simulink model "Elicottero_fuori"  (R2026a)
settings: Solver=VariableStepAuto
values from neighbouring files (symbols this model uses):
  c_alpha = 0.01    [Params_Progetto.m]    (also in Params_Progetto_master.m; parameters.m; parameters_parametrico.m)
  c_beta = 0.01    [Params_Progetto.m]    (also in Params_Progetto_master.m; parameters.m; parameters_parametrico.m)
  eps_p = 0.1    [Params_Progetto.m]    (also in Params_Progetto_master.m; parameters.m; parameters_parametrico.m)
  eps_y = 0.1    [Params_Progetto.m]    (also in Params_Progetto_master.m; parameters.m; parameters_parametrico.m)
  g = 9.81    [Params_Progetto.m]    (also in Params_Progetto_master.m; parameters.m; parameters_parametrico.m)
  h0 = 0.30    (= 0.3)    [Params_Progetto.m]    (also in Params_Progetto_master.m)
  I_b = 0.00023    [Params_Progetto.m]    (also in Params_Progetto_master.m; parameters.m; parameters_parametrico.m)
  J_alpha = 0.012    [Params_Progetto.m]    (also in Params_Progetto_master.m; parameters.m; parameters_parametrico.m)
  J_y = 0.00023    [Params_Progetto.m]    (also in Params_Progetto_master.m; parameters.m; parameters_parametrico.m)
  J_z = 0.00364    [Params_Progetto.m]    (also in Params_Progetto_master.m; parameters.m; parameters_parametrico.m)
  l = 0.2    [Params_Progetto.m]    (also in Params_Progetto_master.m; parameters.m; parameters_parametrico.m)
  m = 0.2    [Params_Progetto.m]    (also in Params_Progetto_master.m; parameters.m; parameters_parametrico.m)
  P0_EKF = diag([ ... (first row only)    [Params_Progetto.m]    (also in Params_Progetto_master.m; parameters.m = diag([1, 1, 1, 1]); parameters_parametrico.m = diag([10, 10, 10, 10]))
  Q_EKF = diag([ ... (first row only)    [Params_Progetto.m]    (also in Params_Progetto_master.m; parameters.m = diag([1e-6, 1e-4, 1e-6, 1e-4]); parameters_parametrico.m = diag([1e-5, 1e-3, 1e-5, 1e-3]))
  R_EKF = diag([ ... (first row only)    [Params_Progetto.m]    (also in Params_Progetto_master.m; parameters.m = diag([std_dev_cam^2, std_dev_cam^2, std_dev_acc^2]); parameters_parametrico.m)
  sigma_acc_sensor = 0.05    [Params_Progetto.m]    (also in Params_Progetto_master.m)
  sigma_alpha_sensor = 0.01    [Params_Progetto.m]    (also in Params_Progetto_master.m)
  sigma_cam_sensor = 0.002    [Params_Progetto.m]    (also in Params_Progetto_master.m = 0.005)
  Ts_Acceler = 1 / 80    (= 0.0125)    [Params_Progetto.m]    (also in Params_Progetto_master.m)
  Ts_EKF = 1/104    (= 0.00961538461538)    [Params_Progetto.m]    (also in Params_Progetto_master.m)
  Ts_ToF_alpha = 1 / 30    (= 0.0333333333333)    [Params_Progetto.m]    (also in Params_Progetto_master.m)
  Ts_Tof_cam = 1/45    (= 0.0222222222222)    [Params_Progetto.m]    (also in Params_Progetto_master.m)
  x0_EKF = [0; 0; 0; 0]    [Params_Progetto.m]    (also in Params_Progetto_master.m; parameters.m; parameters_parametrico.m = [pi/2; 0.2; pi/4; -0.15])
libraries: simulink x2
settings Model: Creator=filin  LastModifiedBy=tomma

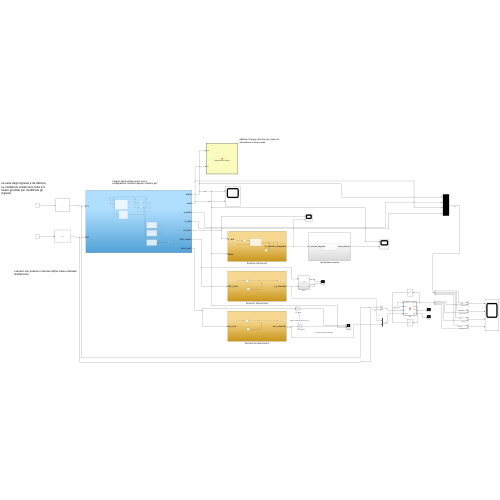
[thumbnail: Simulink's stored preview of the top-level diagram]
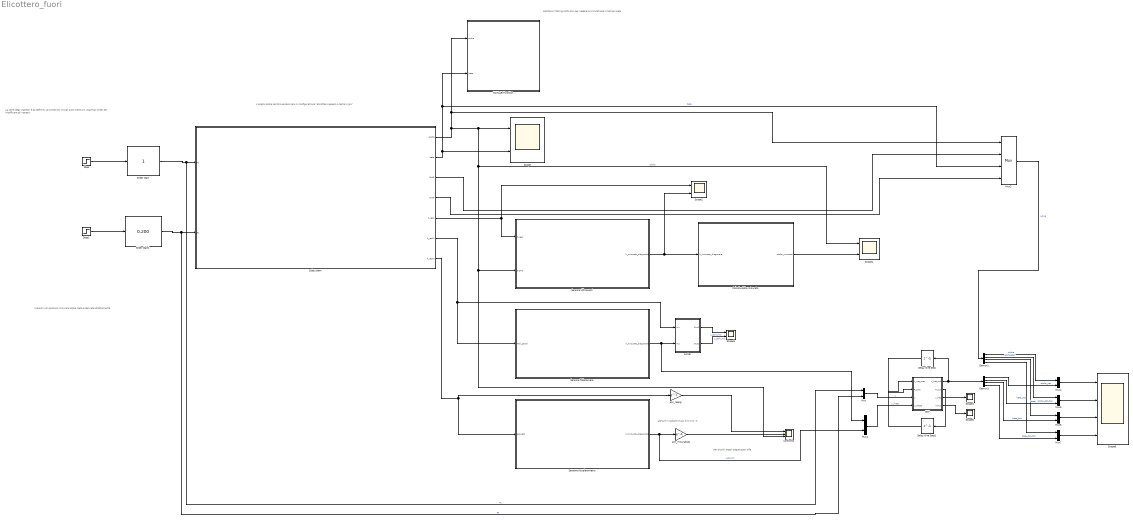
== system Elicottero_fuori ==
  note: alpha è in radianti e acc è in m/s^2
  note: per piccoli angoli segue quasi alfa
  note: L'angolo alpha sembra essere zero in configurazione "elicottero appeso a testa in giù"
  note: Abilitare il Pacing sotto Run per vedere la simulazione in tempo reale
  note: I sensori non possono misurare alpha, beta e derivate direttamente
  note: La serie degli ingressi è da definire,
      | Le condizioni iniziali sono tutte a 0. Usare gli slider per modificare gli ingressi
  Calcola alpha misurato : Subsystem
  Delay One Step : Delay  DelayLength=1  InitialCondition=x0_EKF  SampleTime=Ts_EKF
  Delay One Step1 : Delay  DelayLength=1  InitialCondition=P0_EKF  SampleTime=Ts_EKF
  Demux2 : Demux
  Demux3 : Demux
  EKF : MATLAB Function  TreatAsAtomicUnit=on
  MATLAB Function : MATLAB Function  TreatAsAtomicUnit=on
  Mux{,1,4..7} (6 alike) : Mux  Inputs=2
  Mux2 : Mux
  Scope{,1..3} (4 alike) : Scope  NumInputPorts=2
      Scope settings: ActiveDisplayYMinimum=-0.63060301461050317  ActiveDisplayYMaximum=0.90405934016402656
      Scope1 settings: ActiveDisplayYMinimum=0.070707009259759535  ActiveDisplayYMaximum=0.469619980054257
      Scope2 settings: ActiveDisplayYMinimum=0.074242701385080767  ActiveDisplayYMaximum=0.48624550790168564  DataLoggingVariableName=ScopeData2
      Scope3 settings: ActiveDisplayYMinimum=0.097019421313557869  ActiveDisplayYMaximum=0.17329990637736653  DataLoggingVariableName=ScopeData3
  Scope4 : Scope
      settings: ActiveDisplayYMinimum=-0.80524166083087523  ActiveDisplayYMaximum=1.1715327148927259  DataLoggingVariableName=ScopeData5
  Scope5 : Scope
      settings: ActiveDisplayYMinimum=-0.57698730443451041  ActiveDisplayYMaximum=0.48376451557036515  DataLoggingVariableName=ScopeData6
  Scope6 : Scope  NumInputPorts=4
      settings: ActiveDisplayYMinimum=-0.81874656324729156  ActiveDisplayYMaximum=1.168245552270631  DataLoggingVariableName=ScopeData8
  Sensore Accelerometro : Subsystem
  Sensore Telecamera : Subsystem
  Sensore Ultrasuoni : Subsystem
  Slider Gain : simulink/Math Operations/Slider Gain  gain=1  low=0  high=4
  Slider Gain1 : simulink/Math Operations/Slider Gain  gain=0.200  low=-1  high=1
  Step : Step  InitialValue=1  FinalValue=0  SampleTime=0
  Step1 : Step  InitialValue=1  FinalValue=0  SampleTime=0
  Subsystem : Subsystem
  acc_misurato/g : Gain  Gain=g^-1
  acc_real/g : Gain  Gain=g^-1
  confronto : Scope  NumInputPorts=3
      settings: ActiveDisplayYMinimum=-1.8843706187467704  ActiveDisplayYMaximum=3.0235830228592131  DataLoggingVariableName=ScopeData4
  sorter : Subsystem
  wires:
  Step1/1 -> Slider Gain1/1
  Slider Gain1/1 -> Mux/2, Subsystem/2(F2)  "F2"
  Step/1 -> Slider Gain/1
  Slider Gain/1 -> Mux/1, Subsystem/1(F1)  "F1"
  Subsystem/1(alpha) -> MATLAB Function/1(alpha), Mux2/1, Scope1/1, confronto/3, Sensore Ultrasuoni/2(alpha), Scope/1  "alpha"
  Subsystem/2(beta) -> MATLAB Function/2(beta), Mux2/3, Scope/2  "beta"
  Subsystem/5(h_real) -> Sensore Ultrasuoni/1(h_real), Scope2/1
  Sensore Ultrasuoni/1(h_misurato_diagonale) -> Scope2/2, Calcola alpha misurato/1(h_misurato_diagonale)
  Calcola alpha misurato/1(alpha_misurato) -> Scope1/2
  Subsystem/6(h_real1) -> Sensore Telecamera/1(Tail_coord), sorter/1(In1)
  Sensore Telecamera/1(h_misurato_diagonale) -> Mux1/1, sorter/2(In2)
  sorter/1(Out1) -> Scope3/1  "x_cam_mis"
  sorter/2(Out2) -> Scope3/2  "y_cam_mis"
  Sensore Accelerometro/1(h_misurato_diagonale) -> Mux1/2, acc_misurato/g/1  "acc_mis"
  Subsystem/7(h_real2) -> Sensore Accelerometro/1(acc_real), acc_real/g/1
  acc_real/g/1 -> confronto/1
  acc_misurato/g/1 -> confronto/2
  Delay One Step/1 -> EKF/1(x_hat_prev)
  EKF/2(P_out) -> Delay One Step1/1
  Delay One Step1/1 -> EKF/2(P_prev)
  Mux/1 -> EKF/3(u)  "u"
  Mux1/1 -> EKF/4(y_meas)  "y_meas"
  Subsystem/3(Out3) -> Mux2/2
  Subsystem/4(Out4) -> Mux2/4
  Mux2/1 -> Demux2/1  "x_true"
  EKF/4(innov) -> Scope5/1
  Mux5/1 -> Scope6/2
  Demux3/2 -> Mux5/2  "alpha_dot_hat"
  Demux3/4 -> Mux7/2  "beta_dot_hat"
  Demux2/4 -> Mux7/1  "beta_dot"
  Demux2/3 -> Mux6/1  "beta"
  EKF/1(x_hat_out) -> Demux3/1, Delay One Step/1
  Demux3/3 -> Mux6/2  "beta_hat"
  Demux2/1 -> Mux4/1  "alpha"
  Demux3/1 -> Mux4/2  "alpha_hat"
  Demux2/2 -> Mux5/1  "alpha_dot"
  Mux7/1 -> Scope6/4
  Mux6/1 -> Scope6/3
  Mux4/1 -> Scope6/1
  EKF/3(y_hat) -> Scope4/1

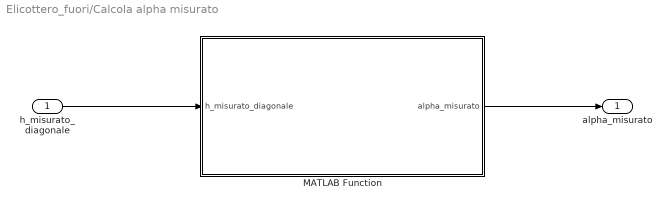
== system Elicottero_fuori/Calcola alpha misurato ==
  h_misurato_diagonale : Inport
  MATLAB Function : MATLAB Function  TreatAsAtomicUnit=on
  alpha_misurato : Outport
  wires:
  h_misurato_diagonale/1 -> MATLAB Function/1(h_misurato_diagonale)
  MATLAB Function/1(alpha_misurato) -> alpha_misurato/1

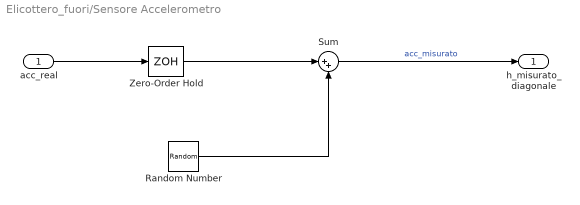
== system Elicottero_fuori/Sensore Accelerometro ==
  acc_real : Inport
  Random Number : RandomNumber  Variance=sigma_acc_sensor^2  Seed=1357  SampleTime=Ts_Acceler
  Sum : Sum  Inputs=|++
  Zero-Order Hold : ZeroOrderHold  SampleTime=Ts_Acceler
  h_misurato_diagonale : Outport
  wires:
  acc_real/1 -> Zero-Order Hold/1
  Zero-Order Hold/1 -> Sum/1
  Random Number/1 -> Sum/2
  Sum/1 -> h_misurato_diagonale/1  "acc_misurato"

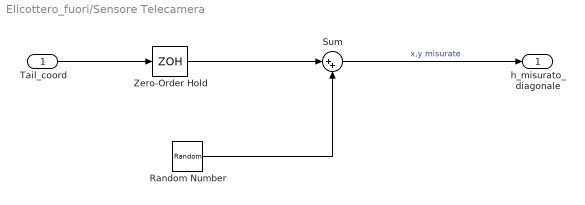
== system Elicottero_fuori/Sensore Telecamera ==
  Tail_coord : Inport
  Random Number : RandomNumber  Variance=sigma_cam_sensor^2  Seed=1357  SampleTime=Ts_Tof_cam
  Sum : Sum  Inputs=|++
  Zero-Order Hold : ZeroOrderHold  SampleTime=Ts_Tof_cam
  h_misurato_diagonale : Outport
  wires:
  Tail_coord/1 -> Zero-Order Hold/1
  Zero-Order Hold/1 -> Sum/1
  Random Number/1 -> Sum/2
  Sum/1 -> h_misurato_diagonale/1  "x,y misurate"

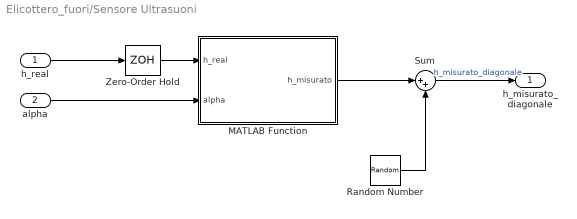
== system Elicottero_fuori/Sensore Ultrasuoni ==
  h_real : Inport
  alpha : Inport  Port=2
  MATLAB Function : MATLAB Function  TreatAsAtomicUnit=on
  Random Number : RandomNumber  Variance=sigma_alpha_sensor^2  Seed=1357  SampleTime=Ts_ToF_alpha
  Sum : Sum  Inputs=|++
  Zero-Order Hold : ZeroOrderHold  SampleTime=Ts_ToF_alpha
  h_misurato_diagonale : Outport
  wires:
  h_real/1 -> Zero-Order Hold/1
  Random Number/1 -> Sum/2
  Sum/1 -> h_misurato_diagonale/1  "h_misurato_diagonale"
  Zero-Order Hold/1 -> MATLAB Function/1(h_real)
  MATLAB Function/1(h_misurato) -> Sum/1
  alpha/1 -> MATLAB Function/2(alpha)

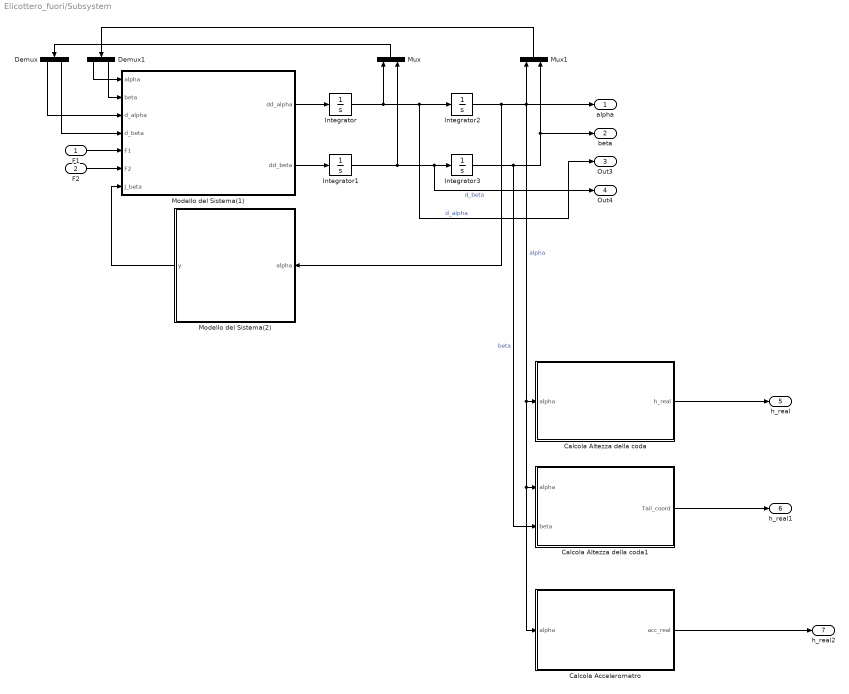
== system Elicottero_fuori/Subsystem ==
  F1 : Inport
  F2 : Inport  Port=2
  Calcola Accelerometro : MATLAB Function  TreatAsAtomicUnit=on
  Calcola Altezza della coda : MATLAB Function  TreatAsAtomicUnit=on
  Calcola Altezza della coda1 : MATLAB Function  TreatAsAtomicUnit=on
  Demux : Demux  Outputs=2
  Demux1 : Demux  Outputs=2
  Integrator : Integrator
  Integrator1 : Integrator
  Integrator2 : Integrator  WrapState=on
  Integrator3 : Integrator  WrapState=on
  Modello del Sistema(1) : MATLAB Function  TreatAsAtomicUnit=on
  Modello del Sistema(2) : MATLAB Function  TreatAsAtomicUnit=on
  Mux : Mux  Inputs=2
  Mux1 : Mux  Inputs=2
  alpha : Outport
  beta : Outport  Port=2
  Out3 : Outport  Port=3
  Out4 : Outport  Port=4
  h_real : Outport  Port=5
  h_real1 : Outport  Port=6
  h_real2 : Outport  Port=7
  wires:
  Demux1/2 -> Modello del Sistema(1)/2(beta)
  Integrator2/1 -> Modello del Sistema(2)/1(alpha), Calcola Accelerometro/1(alpha), Calcola Altezza della coda1/1(alpha), Calcola Altezza della coda/1(alpha), alpha/1, Mux1/1  "alpha"
  Integrator1/1 -> Mux/2, Out4/1, Integrator3/1  "d_beta"
  Mux/1 -> Demux/1
  Demux/2 -> Modello del Sistema(1)/4(d_beta)
  Modello del Sistema(2)/1(y) -> Modello del Sistema(1)/7(J_beta)
  Demux/1 -> Modello del Sistema(1)/3(d_alpha)
  Integrator3/1 -> beta/1, Mux1/2, Calcola Altezza della coda1/2(beta)  "beta"
  Modello del Sistema(1)/1(dd_alpha) -> Integrator/1
  Modello del Sistema(1)/2(dd_beta) -> Integrator1/1
  Demux1/1 -> Modello del Sistema(1)/1(alpha)
  Integrator/1 -> Mux/1, Out3/1, Integrator2/1  "d_alpha"
  Mux1/1 -> Demux1/1
  F2/1 -> Modello del Sistema(1)/6(F2)
  F1/1 -> Modello del Sistema(1)/5(F1)
  Calcola Altezza della coda/1(h_real) -> h_real/1
  Calcola Altezza della coda1/1(Tail_coord) -> h_real1/1
  Calcola Accelerometro/1(acc_real) -> h_real2/1

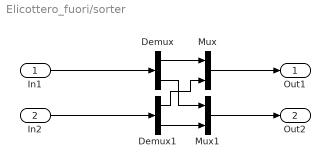
== system Elicottero_fuori/sorter ==
  In1 : Inport
  In2 : Inport  Port=2
  Demux : Demux  Outputs=2
  Demux1 : Demux  Outputs=2
  Mux : Mux  Inputs=2
  Mux1 : Mux  Inputs=2
  Out1 : Outport
  Out2 : Outport  Port=2
  wires:
  Demux/2 -> Mux1/1
  Demux/1 -> Mux/1
  Demux1/1 -> Mux/2
  In1/1 -> Demux/1
  Mux1/1 -> Out2/1
  In2/1 -> Demux1/1
  Demux1/2 -> Mux1/2
  Mux/1 -> Out1/1

== matlab function Elicottero_fuori/Subsystem/Calcola Accelerometro ==
  data: alpha input; acc_real output; g parameter
function acc_real = Compute_Accelerometer(alpha, g)

%%Si assume un accelerometro monoassiale solidale al corpo,
% orientato in modo da misurare la componente della gravità dovuta al pitch.

acc_real = g * sin(alpha);

%acc_real = -g * sin(alpha); quale usiamo?
end

== matlab function Elicottero_fuori/EKF ==
  data: x_hat_prev input; P_prev input; u input; x_hat_out output; y_meas input; P_out output; Ts_EKF parameter; Q_EKF parameter; R_EKF parameter; J_alpha parameter; J_y parameter; J_z parameter; I_b parameter; m parameter; l parameter; g parameter; c_alpha parameter; c_beta parameter; eps_p parameter; eps_y parameter; y_hat output; innov output
function [x_hat_out, P_out, y_hat, innov] = EKF(x_hat_prev, P_prev, u, y_meas, Ts_EKF, Q_EKF, R_EKF, J_alpha, J_y, J_z, I_b, m, l, g, c_alpha, c_beta, eps_p, eps_y)
% EKF
%
% Ingressi:
%   x_hat_prev = [alpha_hat; d_alpha_hat; beta_hat; d_beta_hat]
%   P_prev     = matrice 4x4 della covarianza precedente
%   u          = [F1; F2]
%   y_meas     = [x_cam_mis; y_cam_mis; acc_mis]
%
% Uscite:
%   x_hat_out  = stato corretto al passo corrente
%   P_out      = covarianza corretta al passo corrente

% ============================================================
% 1. Estrazione ingressi
% ============================================================

F1 = u(1);
F2 = u(2);

alpha   = x_hat_prev(1);
d_alpha = x_hat_prev(2);
beta    = x_hat_prev(3);
d_beta  = x_hat_prev(4);

% ============================================================
% 2. Modello dinamico continuo dell'elicottero
%    x_dot = f(x,u)
% ============================================================

J_beta = J_y*sin(alpha)^2 + (J_z + m*l^2)*cos(alpha)^2 + I_b;

dd_alpha = ( ...
    - c_alpha*d_alpha ...
    - m*g*l*sin(alpha) ...
    + l*F1*cos(beta) ...
    + eps_p*l*F2*sin(beta) ...
            ) / J_alpha;

dd_beta = ( ...
    - c_beta*d_beta ...
    + l*F2*cos(alpha) ...
    + eps_y*l*F1*sin(alpha) ...
          ) / J_beta;

f = [
    d_alpha;
    dd_alpha;
    d_beta;
    dd_beta
];

% ============================================================
% 3. Predizione discreta tramite Eulero
%    x(k|k-1) = x(k-1|k-1) + Ts*f(x,u)
% ============================================================

x_pred = x_hat_prev + Ts_EKF*f;

% ============================================================
% 4. Jacobiana continua A_c = df/dx
% ============================================================

Kgeom = J_z + m*l^2;

dJbeta_dalpha = 2*sin(alpha)*cos(alpha)*(J_y - Kgeom);

% Derivate di dd_alpha
d_ddalpha_d_alpha = -m*g*l*cos(alpha) / J_alpha;

d_ddalpha_d_dalpha = -c_alpha / J_alpha;

d_ddalpha_d_beta = ( ...
    -l*F1*sin(beta) ...
    + eps_p*l*F2*cos(beta) ...
    ) / J_alpha;

d_ddalpha_d_dbeta = 0;

% Derivate di dd_beta
N_beta = ...
    - c_beta*d_beta ...
    + l*F2*cos(alpha) ...
    + eps_y*l*F1*sin(alpha);

dNbeta_dalpha = ...
    - l*F2*sin(alpha) ...
    + eps_y*l*F1*cos(alpha);

d_ddbeta_d_alpha = ...
    (dNbeta_dalpha*J_beta - N_beta*dJbeta_dalpha) / (J_beta^2);

d_ddbeta_d_dalpha = 0;

d_ddbeta_d_beta = 0;

d_ddbeta_d_dbeta = -c_beta / J_beta;

A_c = [
    0,                 1,                  0,                0;
    d_ddalpha_d_alpha, d_ddalpha_d_dalpha, d_ddalpha_d_beta, d_ddalpha_d_dbeta;
    0,                 0,                  0,                1;
    d_ddbeta_d_alpha,  d_ddbeta_d_dalpha,  d_ddbeta_d_beta,  d_ddbeta_d_dbeta
];

% Jacobiana discreta
F_k = eye(4) + Ts_EKF*A_c;

% Predizione covarianza
P_pred = F_k*P_prev*F_k' + Q_EKF;

% Simmetrizzazione numerica
P_pred = (P_pred + P_pred')/2;

% ============================================================
% 5. Modello di misura camera + accelerometro
%
% y = h(x) + v
%
% y_meas = [
%   x_cam;
%   y_cam;
%   acc
% ]
% ============================================================

alpha_p = x_pred(1);
beta_p  = x_pred(3);

h = [
    l*cos(alpha_p)*cos(beta_p);
    l*cos(alpha_p)*sin(beta_p);
    g*sin(alpha_p)
];
y_hat = h;

% ============================================================
% 6. Jacobiana della misura H = dh/dx
% ============================================================

H = [
    -l*sin(alpha_p)*cos(beta_p), 0, -l*cos(alpha_p)*sin(beta_p), 0;
    -l*sin(alpha_p)*sin(beta_p), 0,  l*cos(alpha_p)*cos(beta_p), 0;
     g*cos(alpha_p),             0,  0,                          0
];

% ============================================================
% 7. Correzione EKF
% ============================================================

innov = y_meas - h;

S = H*P_pred*H' + R_EKF;

K = P_pred*H'/S;

x_hat_out = x_pred + K*innov;

% Riporto beta in [-pi, pi]
x_hat_out(3) = atan2(sin(x_hat_out(3)), cos(x_hat_out(3)));

%% come l'abbiamo vista a lezione 
P_out = P_pred - K*S*K';
P_out = (P_out + P_out')/2;
% Simmetrizzazione numerica finale
P_out = (P_out + P_out')/2;

end

== matlab function Elicottero_fuori/Subsystem/Modello del Sistema(2) ==
  data: alpha input; y output; J_y parameter; J_z parameter; m parameter; l parameter; I_b parameter
function y = Aggiorna_J_beta(alpha, J_y, J_z, m, l, I_b)

J_beta = J_y * (sin(alpha) ^ 2) + (J_z + m * l ^ 2) * (cos(alpha)) ^ 2 + I_b; 

y = J_beta;

== matlab function Elicottero_fuori/Subsystem/Modello del Sistema(1) ==
  data: alpha input; beta input; dd_alpha output; d_alpha input; d_beta input; F1 input; F2 input; J_beta input; dd_beta output; c_alpha parameter; m parameter; g parameter; l parameter; eps_p parameter; J_alpha parameter; c_beta parameter; eps_y parameter
function [dd_alpha, dd_beta] = Helicopter_Helicopter(alpha, beta, d_alpha, d_beta, F1, F2, J_beta, c_alpha, m, g, l, eps_p, J_alpha, c_beta, eps_y)

dd_alpha        = (- c_alpha * d_alpha - m * g * l * sin(alpha) + l * F1...
                    * cos(beta) + eps_p * l * F2 * sin(beta)) / J_alpha;

dd_beta        = (- c_beta * d_beta + l * F2 * cos(alpha) + eps_y * l * F1...
                    * sin(alpha)) / J_beta;

== matlab function Elicottero_fuori/MATLAB Function ==
  data: alpha input; beta input
function Disegna_Elicottero_Realtime(alpha, beta)
    % Definisce i dati come persistenti per non ricreare la finestra a ogni step
    persistent f h_pitch h_yaw l;
    
    if isempty(f)
        l = 0.2; % Lunghezza braccio
        f = figure('Name', 'Simulatore Elicottero 2-DoF');
        
        % Subplot 1: Vista Laterale (Pitch)
        subplot(2,1,1);
        hold on; grid on; axis equal;
        axis([-0.3 0.3 -0.3 0.3]);
        plot([0 0], [-0.3 0], 'k', 'LineWidth', 3); % Perno base
        h_pitch = plot([0 0], [0 0], 'b-o', 'LineWidth', 4, 'MarkerSize', 10);
        title('Vista Laterale - Pitch (\alpha)');
        
        % Subplot 2: Vista dall'Alto (Yaw)
        subplot(2,1,2);
        hold on; grid on; axis equal;
        axis([-0.3 0.3 -0.3 0.3]);
        plot(0, 0, 'k+', 'MarkerSize', 10); % Centro
        h_yaw = plot([0 0], [0 0], 'r-o', 'LineWidth', 4, 'MarkerSize', 10);
        title('Vista dall''Alto - Yaw (\beta)');
    end
    
    % Aggiornamento delle coordinate geometriche
    
    % Pitch: rotazione nel piano verticale X-Z
    % Sfasamento di pi (180 gradi) per posizionare il braccio a sinistra a alpha = 0
    alpha_grafico = alpha + pi; 
    
    x_p = l * cos(alpha_grafico);
    z_p = l * sin(alpha_grafico);
    set(h_pitch, 'XData', [0 x_p], 'YData', [0 z_p]);
        
    % Yaw: rotazione nel piano orizzontale X-Y
    beta_grafico = beta + pi; % Trasla anche lo yaw per coerenza visiva
    x_y = l * cos(beta_grafico);
    y_y = l * sin(beta_grafico);
    set(h_yaw, 'XData', [0 x_y], 'YData', [0 y_y]);
    
    drawnow limitrate; % Forza l'aggiornamento grafico
end

== matlab function Elicottero_fuori/Sensore Ultrasuoni/MATLAB Function ==
  data: h_misurato output; h_real input; alpha input
function h_misurato =  Wenglor_U1KT001(h_real, alpha)

h_misurato = h_real / cos(alpha);

y = h_misurato;

== matlab function Elicottero_fuori/Subsystem/Calcola Altezza della coda ==
  data: alpha input; h_real output; l parameter; h0 parameter
function h_real = Compute_Tail_height(alpha, l, h0)

% Sensore ultrasuoni sotto il muso.
% Misura la distanza verticale del muso dal tavolo.
%
% Modello:
% y_alpha = h0 + l_s_alpha * sin(alpha)

h_real = h0 - l * sin(alpha);

end

== matlab function Elicottero_fuori/Calcola alpha misurato/MATLAB Function ==
  data: h_misurato_diagonale input; alpha_misurato output; l parameter; h0 parameter
function alpha_misurato = compute_alpha(h_misurato_diagonale, l, h0)

    % Metodo dell'angolo aggiunto per l'inversione analitica:
    % y_meas * cos(alpha) + l * sin(alpha) = H0
    
    R = sqrt(h_misurato_diagonale^2 + l^2);
    phi = atan2(l, h_misurato_diagonale);
    
    % Controllo di sicurezza per l'argomento dell'arcocoseno
    arg_acos = h0 / R;
    if arg_acos > 1
        arg_acos = 1;
    elseif arg_acos < -1
        arg_acos = -1;
    end
    
    % Calcolo dell'angolo invertito
    % Scegliamo la soluzione geometricamente coerente con il quadrante operativo
    alpha_misurato = phi - acos(arg_acos);
end

== matlab function Elicottero_fuori/Subsystem/Calcola Altezza della coda1 ==
  data: alpha input; beta input; Tail_coord output; l parameter; h0 parameter
function Tail_coord = Compute_Tail_coordinates(alpha, beta, l, h0)

x = l * cos(alpha) * cos(beta);
y = l * cos(alpha) * sin(beta);

Tail_coord = [x ; y]; 

end
